simulink model "Active_skyhook"  (R2018a)
settings: Solver=VariableStepAuto  StartTime=0.0  StopTime=5  RelTol=1e-3
values from neighbouring files (symbols this model uses):
  A = [0 1 0 0 ... (first row only)    [Bounce_controll.m]    (also in Workspace.m = [0 1 0 0;-ks/ms 0 ks/ms 0;0 0 0 1;ks/mp 0 -(ks+kp)/mp -cp/mp)
  B = [0 0 0 0 ... (first row only)    [Bounce_controll.m]    (also in Workspace.m = [0 0 0;1/ms 0 0;0 0 0;-1/mp kp/mp cp/mp])
  C = [0 1 0 0 ... (first row only)    [Bounce_controll.m]    (also in Workspace.m = [1 0 0 0])
  Cx = 4e6    (= 4000000)    [Bounce_controll.m]
  Cz = 24e3    (= 24000)    [Bounce_controll.m]
  D = [0 0 0 0 ... (first row only)    [Bounce_controll.m]    (also in Workspace.m = [0 0 0])
  L = 6    [Bounce_controll.m]    (also in H_inf_ctrl.m)
  sinfreq = testHZ*2*pi    (= 6.28318530718)    [Bounce_controll.m]
settings Model: Creator=c_s  LastModifiedBy=c_s

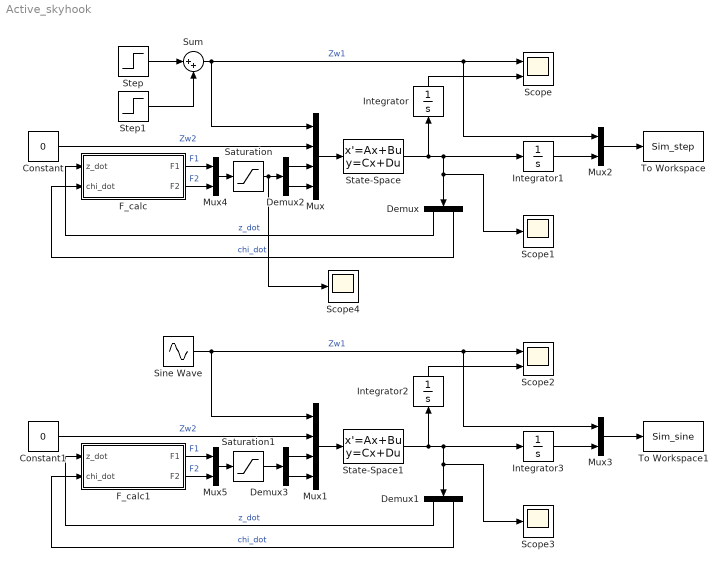
== system Active_skyhook ==
  Constant : Constant  Value=0
  Constant1 : Constant  Value=0
  Demux{,1..3} (4 alike) : Demux  Outputs=2
  F_calc : Subsystem
  F_calc1 : Subsystem
  Integrator{,1..3} (4 alike) : Integrator
  Mux : Mux
  Mux1 : Mux
  Mux{2..5} (4 alike) : Mux  Inputs=2
  Saturation : Saturate  UpperLimit=10e3  LowerLimit=-10e3
  Saturation1 : Saturate  UpperLimit=10e3  LowerLimit=-10e3
  Scope : Scope  NumInputPorts=2
  Scope1 : Scope
  Scope2 : Scope  NumInputPorts=2
  Scope3 : Scope
  Scope4 : Scope
  Sine Wave : Sin  Amplitude=0.01  Frequency=sinfreq  SampleTime=0
  State-Space : StateSpace  A=A  B=B  C=C  D=D  InitialCondition=0
  State-Space1 : StateSpace  A=A  B=B  C=C  D=D  InitialCondition=0
  Step : Step  Time=0  After=0.03  SampleTime=0
  Step1 : Step  After=-0.03  SampleTime=0
  Sum : Sum  Inputs=|++
  To Workspace : ToWorkspace  VariableName=Sim_step  SaveFormat=Structure With Time  SampleTime=-1
  To Workspace1 : ToWorkspace  VariableName=Sim_sine  SaveFormat=Structure With Time  SampleTime=-1
  wires:
  Mux/1 -> State-Space/1
  Sum/1 -> Mux/1, Mux2/1, Scope/1  "Zw1"
  Step/1 -> Sum/1
  Constant/1 -> Mux/2  "Zw2"
  Step1/1 -> Sum/2
  F_calc/1(F1) -> Mux4/1  "F1"
  Demux/1 -> F_calc/1(z_dot)  "z_dot"
  Demux/2 -> F_calc/2(chi_dot)  "chi_dot"
  State-Space/1 -> Integrator1/1, Scope1/1, Demux/1, Integrator/1
  F_calc/2(F2) -> Mux4/2  "F2"
  Integrator/1 -> Scope/2
  Mux2/1 -> To Workspace/1
  Integrator1/1 -> Mux2/2
  Mux4/1 -> Saturation/1
  Saturation/1 -> Scope4/1, Demux2/1
  Demux2/1 -> Mux/3
  Demux2/2 -> Mux/4
  Demux3/2 -> Mux1/4
  Demux3/1 -> Mux1/3
  Saturation1/1 -> Demux3/1
  Mux5/1 -> Saturation1/1
  Integrator3/1 -> Mux3/2
  Mux3/1 -> To Workspace1/1
  Integrator2/1 -> Scope2/2
  F_calc1/2(F2) -> Mux5/2  "F2"
  State-Space1/1 -> Integrator2/1, Demux1/1, Scope3/1, Integrator3/1
  Demux1/2 -> F_calc1/2(chi_dot)  "chi_dot"
  Demux1/1 -> F_calc1/1(z_dot)  "z_dot"
  F_calc1/1(F1) -> Mux5/1  "F1"
  Constant1/1 -> Mux1/2  "Zw2"
  Sine Wave/1 -> Scope2/1, Mux3/1, Mux1/1  "Zw1"
  Mux1/1 -> State-Space1/1

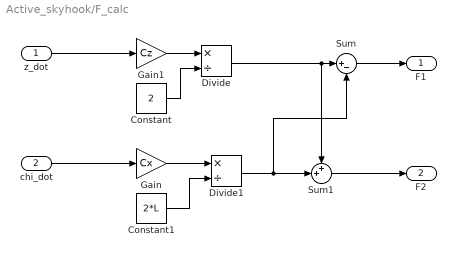
== system Active_skyhook/F_calc ==
  z_dot : Inport
  chi_dot : Inport  Port=2
  Constant : Constant  Value=2
  Constant1 : Constant  Value=2*L
  Divide : Product  Inputs=*/
  Divide1 : Product  Inputs=*/
  Gain : Gain  Gain=Cx
  Gain1 : Gain  Gain=Cz
  Sum : Sum  Inputs=|+-
  Sum1 : Sum  Inputs=++|
  F1 : Outport
  F2 : Outport  Port=2
  wires:
  Sum/1 -> F1/1
  Gain/1 -> Divide1/1
  Divide/1 -> Sum1/1, Sum/1
  Sum1/1 -> F2/1
  Constant/1 -> Divide/2
  Gain1/1 -> Divide/1
  Constant1/1 -> Divide1/2
  Divide1/1 -> Sum/2, Sum1/2
  z_dot/1 -> Gain1/1
  chi_dot/1 -> Gain/1

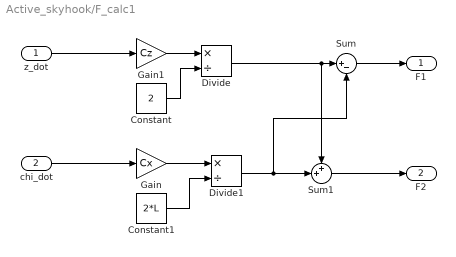
== system Active_skyhook/F_calc1 ==
  z_dot : Inport
  chi_dot : Inport  Port=2
  Constant : Constant  Value=2
  Constant1 : Constant  Value=2*L
  Divide : Product  Inputs=*/
  Divide1 : Product  Inputs=*/
  Gain : Gain  Gain=Cx
  Gain1 : Gain  Gain=Cz
  Sum : Sum  Inputs=|+-
  Sum1 : Sum  Inputs=++|
  F1 : Outport
  F2 : Outport  Port=2
  wires:
  chi_dot/1 -> Gain/1
  z_dot/1 -> Gain1/1
  Divide1/1 -> Sum1/2, Sum/2
  Constant1/1 -> Divide1/2
  Gain1/1 -> Divide/1
  Constant/1 -> Divide/2
  Sum1/1 -> F2/1
  Divide/1 -> Sum/1, Sum1/1
  Gain/1 -> Divide1/1
  Sum/1 -> F1/1
